simulink model "r4_pfb_fir"  (Simulink 7.0)
settings: Solver=FixedStepDiscrete  SolverMode=SingleTasking  StartTime=0.0  StopTime=10.0  RelTol=1e-3
undefined symbols (not defined in the file): pfb_coefs
libraries: xbsIndex_r4 x385, xps_library x1
(part 11 of 27)

== system r4_pfb_fir/fir_2/fir_tap_6 ==
  data_in : Inport  OutDataType=sfix(16)  OutScaling=2^0
  sum_in : Inport  Port=2  OutDataType=sfix(16)  OutScaling=2^0
  sync_in : Inport  Port=3  OutDataType=sfix(16)  OutScaling=2^0
  fir_coef : Subsystem  mask(FIR Filter Coefficient Generator){coef=[1.30229478472013e-005;3.90815624059165e-005;6.51573367774649e-005;9.12505128142159e-005;0.000117361332654004;0.000143490038707315;0.000169636873644433;0.000195802080382638;0.000221985902073233;0.000248188582088693;0.00027441036400972;0.000300651491612275;0.00032691220885466;0.000353192759864432;0.00037949338892544;0.000405814340464771;0.000432155859039685;0.000458518189324518;0.000484901576097635;0.000511306264228219;0.00053773249866318;0.000564180524413982;0.000590650586543436;0.000617142930152563;0.000643657800367275;0.000670195442325197;0.000696756101162392;0.00072334002200008;0.000749947449931329;0.000776578630007802;0.000803233807226332;0.000829913226515637;0.00085661713272294;0.000883345770600572;0.000910099384792634;0.000936878219821494;0.000963682520074419;0.000990512529790111;0.00101736849304526;0.00104425065374103;0.00107115925558966;0.00109809454210086;0.00112505675656834;0.00115204614205629;0.0011790629413858;0.00120610739712138;0.00123317975155729;0.00126028024670401;0.00128740912427467;0.0013145666256714;0.00134175299197172;0.00136896846391498;0.00139621328188859;0.00142348768591449;0.00145079191563545;0.00147812621030134;0.0015054908087556;0.00153288594942139;0.00156031187028796;0.00158776880889696;0.00161525700232871;0.00164277668718846;0.00167032809959269;0.00169791147515534;0.00172552704897407;0.00175317505561652;0.00178085572910654;0.00180856930291045;0.00183631600992321;0.00186409608245468;0.00189190975221584;0.001919757250305;0.00194763880719397;0.00197555465271432;0.00200350501604353;0.00203149012569121;0.00205951020948525;0.00208756549455806;0.00211565620733274;0.00214378257350922;0.00217194481805049;0.00220014316516874;0.00222837783831153;0.002256649060148;0.00228495705255503;0.00231330203660339;0.00234168423254391;0.00237010385979366;0.00239856113692212;0.00242705628163739;0.00245558951077227;0.0024841610402705;0.00251277108517291;0.00254141985960361;0.00257010757675613;0.00259883444887969;0.00262760068726523;0.00265640650223175;0.00268525210311237;0.00271413769824061;0.00274306349493657;0.00277202969949308;0.00280103651716193;0.00283008415214012;0.00285917280755598;0.00288830268545549;0.00291747398678844;0.00294668691139467;0.00297594165799033;0.00300523842415407;0.00303457740631335;0.00306395879973069;0.00309338279848989;0.00312284959548233;0.00315235938239325;0.00318191234968804;0.00321150868659852;0.00324114858110932;0.00327083221994408;0.00330055978855185;0.00333033147109343;0.00336014745042765;0.00339000790809786;0.00341991302431814;0.0034498629779598;0.00347985794653768;0.00350989810619665;0.00353998363169792;0.0035701146964056;0.00360029147227299;0.00363051412982916;0.00366078283816534;0.00369109776492143;0.00372145907627252;0.00375186693691537;0.00378232151005492;0.00381282295739088;0.00384337143910425;0.00387396711384388;0.00390461013871314;0.00393530066925641;0.00396603885944579;0.00399682486166768;0.00402765882670945;0.0040585409037462;0.00408947124032728;0.00412044998236316;0.00415147727411206;0.00418255325816677;0.00421367807544131;0.00424485186515788;0.00427607476483351;0.00430734691026696;0.00433866843552555;0.00437003947293203;0.00440146015305152;0.00443293060467832;0.00446445095482291;0.00449602132869889;0.00452764184970998;0.00455931263943696;0.00459103381762476;0.00462280550216948;0.00465462780910543;0.00468650085259228;0.0047184247449021;0.00475039959640664;0.00478242551556433;0.00481450260890759;0.00484663098103001;0.00487881073457359;0.00491104197021601;0.00494332478665798;0.00497565928061048;0.00500804554678217;0.00504048367786674;0.00507297376453033;0.00510551589539899;0.0051381101570461;0.00517075663397987;0.00520345540863088;0.00523620656133964;0.0052690101703441;0.00530186631176739;0.00533477505960533;0.00536773648571416;0.00540075065979826;0.00543381764939783;0.00546693751987671;0.00550011033441016;0.00553333615397264;0.00556661503732576;0.00559994704100609;0.00563333221931314;0.00566677062429732;0.0057002623057479;0.00573380731118106;0.00576740568582796 ...(+15802 chars)], n_bits_c=9, bin_pt_c=8, use_bram=on}
      mask prompts: coef "Tap Coefficient(s)"; n_bits_c "Number of Coefficient Bits"; bin_pt_c "Coefficient Binary Point"; use_bram "Use BRAM for Coefficients"
      mask help: A Finite Impluse Response filter coefficient generator. This FIR filter coefficient generator outputs real coefficients. It can output one coefficient or cycle through a vector of coefficients for WOLA (Weighted OverLap Add) FIR filters.
      settings: AttributesFormatString=1024 coefs in bram
      mask Help:
      | <pre>
      | Description::
      | 
      | A Finite Impluse Response filter coefficient generator.
      | This FIR filter coefficient generator outputs real coefficients.
      | It can output one coefficient or cycle through a vector of coefficients for WOLA
      | (Weighted OverLap Add) FIR filters.
      | 
      | Mask Parameters::
      | 
      | Tap Coefficiant(s) (coef): The coefficient(s) to output.  For a "regular" FIR filter, this will be a
      | single number.  For a WOLA (Weighted OverLap Add) filter, this will be a vector of numbers.
      | These should be specified as doubles.   They will be rounded and saturated according to the
      | specified number of bits (n_bits_c) and binary point (bin_pt_c).
      | 
      | Number of Coefficient Bits (n_bits_c): The number of bits used for the fixed point binary
      | representation of the coefficient(s).
      | 
      | Coefficient Binary Point (bin_pt_c): The binary point of the fixed point binary representation
      | of the coefficient(s).
      | 
      | Use BRAM for Coefficients (use_bram): Check this checkbox to store the coefficients in BRAM.
      | If unchecked, the coefficients will be stored in distributed memory (i.e. slices).
      | This is only relevant is length(coef) is greater than 1; otherwise, a constant block is used.
      | </pre>
  fir_core : Subsystem  mask(FIR Filter Core){delay=0, n_bits_d=8, bin_pt_d=7, n_bits_s=17, bin_pt_s=15, use_bram=off, mult_latency=3, add_latency=1, add_bypass=off}
      mask prompts: delay "Tap Delay"; n_bits_d "Number of Data Bits"; bin_pt_d "Data Binary Point"; n_bits_s "Number of Sum Bits"; bin_pt_s "Sum Binary Point"; use_bram "Use BRAM for Delay"; mult_latency "Multiplier Latency"; add_latency "Adder Latency"; add_bypass "Bypass Adder"
      mask help: A Finite Impluse Response Filter core with complex inputs and real coefficients. This FIR filter core does not have provisions for folding the input sequence to improve multiplier efficiency, so it is suboptimal for "regular" (i.e. non-WOLA) FIR filters. It is intended primarily for WOLA (Weighted OverLap Add) FIR filters.
      settings: AttributesFormatString=delay 0 in slr
      mask Help:
      | <pre>
      | Description::
      | 
      | A Finite Impluse Response Filter core with complex inputs and real coefficients.
      | 
      | This Finite Impluse Response Filter core is designed to be paired with a FIR Coefficient Generator
      | to form a FIR filter tap.  This FIR filter core does not have provisions for folding the input
      | sequence to improve multiplier efficiency, so it is suboptimal for "regular" (i.e. non-WOLA)
      | FIR filters.  It is intended primarily for WOLA (Weighted OverLap Add) FIR filters.
      | 
      | Mask Parameters::
      | 
      | Tap Delay (delay):  The inter-tap delay (the N in "z^-N").  For a regular FIR filter, this will be 1.
      | 
      | Number of Data Bits (n_bits_d): The number of bits for real/imaginary components of the data.
      | 
      | Data Binary Point (bin_pt_d): The binary point for real/imaginary components of the data.
      | 
      | Number of Sum Bits (n_bits_s): Specifies the width of the sum (overflow wraps).
      | 
      | Sum Binary Point (bin_pt_s): Specifies the binary point of the sum (quantization truncates).
      | 
      | Use BRAM for Delay (use_bram): Check this checkbox to implement the delay using BRAM.
      | If unchecked, the delay will be implemented using SLR16 elements (i.e. slices).
      | 
      | Multiplier Latency (mult_latency): Latency to use for the underlying multiplier.
      | 
      | Adder Latency (add_latency): Latency to use for the underlying adder.
      | 
      | Adder Bypass (add_bypass): Check this checkbox to bypass the adder.
      | Typically used for the first tap of a multi-tap FIR filter.
      | </pre>
  data_out : Outport  OutDataType=sfix(16)  OutScaling=2^0
  sum_out : Outport  Port=2  OutDataType=sfix(16)  OutScaling=2^0
  sync_out : Outport  Port=3  OutDataType=sfix(16)  OutScaling=2^0
  wires:
  fir_core/3(sync_out) -> sync_out/1
  fir_core/2(sum_out) -> sum_out/1
  fir_core/1(data_out) -> data_out/1
  sync_in/1 -> fir_coef/3(sync_in)
  sum_in/1 -> fir_coef/2(sum_in)
  data_in/1 -> fir_coef/1(data_in)
  fir_coef/4(sync_out) -> fir_core/4(sync_in)
  fir_coef/3(coef) -> fir_core/3(coef)
  fir_coef/2(sum_out) -> fir_core/2(sum_in)
  fir_coef/1(data_out) -> fir_core/1(data_in)

== system r4_pfb_fir/fir_1/fir_quantize/c_to_ri ==
  c : Inport  OutDataType=sfix(16)  OutScaling=2^0
  force_im : xbsIndex_r4/Reinterpret  force_arith_type=on  arith_type="Signed  (2's comp)"  force_bin_pt=on  bin_pt=15  block_type=reinterpret
      settings: infoedit="Changes signal type without altering the binary representation.   You can changed the signal between signed and unsigned, and relocate the binary point.<P><P>Hardware notes: In hardware this block costs nothing.<P><P>Example:  Suppose the input is 6 bits wide, signed, with 2 fractional bits, and the output is forced to unsigned with 0 fractional bits.  Then an input of -2.0 (1110.00 in binary 2's complement) becomes an output of 56 (111000 in binary)."  block_version=10.1.3
  force_re : xbsIndex_r4/Reinterpret  force_arith_type=on  arith_type="Signed  (2's comp)"  force_bin_pt=on  bin_pt=15  block_type=reinterpret
      settings: infoedit="Changes signal type without altering the binary representation.   You can changed the signal between signed and unsigned, and relocate the binary point.<P><P>Hardware notes: In hardware this block costs nothing.<P><P>Example:  Suppose the input is 6 bits wide, signed, with 2 fractional bits, and the output is forced to unsigned with 0 fractional bits.  Then an input of -2.0 (1110.00 in binary 2's complement) becomes an output of 56 (111000 in binary)."  block_version=10.1.3
  slice_im : xbsIndex_r4/Slice  nbits=17  boolean_output=off  mode=Lower Bit Location + Width  bit1=0  base1=MSB of Input  bit0=0  base0=LSB of Input  dbl_ovrd=off  block_type=slice
      settings: infoedit="Extracts a given range of bits from each input sample and presents it at the output.  The output type is ordinarily unsigned with binary point at zero, but can be Boolean when the slice is one bit wide.<P><P>Hardware notes: In hardware this block costs nothing."  block_version=10.1.3
  slice_re : xbsIndex_r4/Slice  nbits=17  boolean_output=off  mode=Upper Bit Location + Width  bit1=0  base1=MSB of Input  bit0=0  base0=LSB of Input  dbl_ovrd=off  block_type=slice
      settings: infoedit="Extracts a given range of bits from each input sample and presents it at the output.  The output type is ordinarily unsigned with binary point at zero, but can be Boolean when the slice is one bit wide.<P><P>Hardware notes: In hardware this block costs nothing."  block_version=10.1.3
  re : Outport  OutDataType=sfix(16)  OutScaling=2^0
  im : Outport  Port=2  OutDataType=sfix(16)  OutScaling=2^0
  wires:
  slice_re/1 -> force_re/1
  slice_im/1 -> force_im/1
  force_re/1 -> re/1
  force_im/1 -> im/1
  c/1 -> slice_re/1, slice_im/1

== system r4_pfb_fir/fir_1/fir_quantize/ri_to_c ==
  re : Inport  OutDataType=sfix(16)  OutScaling=2^0
  im : Inport  Port=2  OutDataType=sfix(16)  OutScaling=2^0
  concat : xbsIndex_r4/Concat  num_inputs=2  dbl_ovrd=off  block_type=concat
      settings: block_version=10.1.3
  force_im : xbsIndex_r4/Reinterpret  force_arith_type=on  arith_type=Unsigned  force_bin_pt=on  bin_pt=0  block_type=reinterpret
      settings: infoedit="Changes signal type without altering the binary representation.   You can changed the signal between signed and unsigned, and relocate the binary point.<P><P>Hardware notes: In hardware this block costs nothing.<P><P>Example:  Suppose the input is 6 bits wide, signed, with 2 fractional bits, and the output is forced to unsigned with 0 fractional bits.  Then an input of -2.0 (1110.00 in binary 2's complement) becomes an output of 56 (111000 in binary)."  block_version=10.1.3
  force_re : xbsIndex_r4/Reinterpret  force_arith_type=on  arith_type=Unsigned  force_bin_pt=on  bin_pt=0  block_type=reinterpret
      settings: infoedit="Changes signal type without altering the binary representation.   You can changed the signal between signed and unsigned, and relocate the binary point.<P><P>Hardware notes: In hardware this block costs nothing.<P><P>Example:  Suppose the input is 6 bits wide, signed, with 2 fractional bits, and the output is forced to unsigned with 0 fractional bits.  Then an input of -2.0 (1110.00 in binary 2's complement) becomes an output of 56 (111000 in binary)."  block_version=10.1.3
  c : Outport  OutDataType=sfix(16)  OutScaling=2^0
  wires:
  im/1 -> force_im/1
  concat/1 -> c/1
  re/1 -> force_re/1
  force_im/1 -> concat/2
  force_re/1 -> concat/1
